simulink model "speed_modelo_motor_frenado_con_codigoC"  (R2022b)
settings: Solver=VariableStepAuto  StartTime=0.0  StopTime=5  FixedStep=0.01  MaxStep=0.00005  RelTol=1e-3
undefined symbols (not defined in the file): frec_max_f_freno, frec_motor_max_f, frecuencia, frecuencia_freno, FuerzaX_acel, FuerzaX_freno, FuerzaY_acel, Ipeak, L, mass, pole_length, r, slip, slip_freno, vel_motor_max_f, vel_motor_max_f_freno
libraries: slpidlib x2, pi_con_C x1, eePowerMeasurement x1
settings Model: Creator=mique  LastModifiedBy=mique
settings SolverCC: ZeroCrossAlgorithm=Adaptive
settings DebuggingCC: IgnoredZcDiagnostic=none

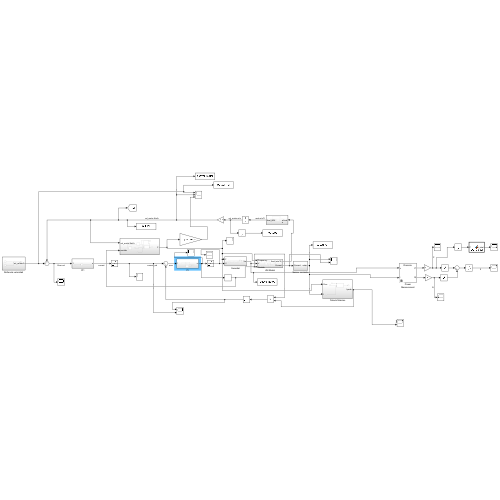
[thumbnail: Simulink's stored preview of the top-level diagram]
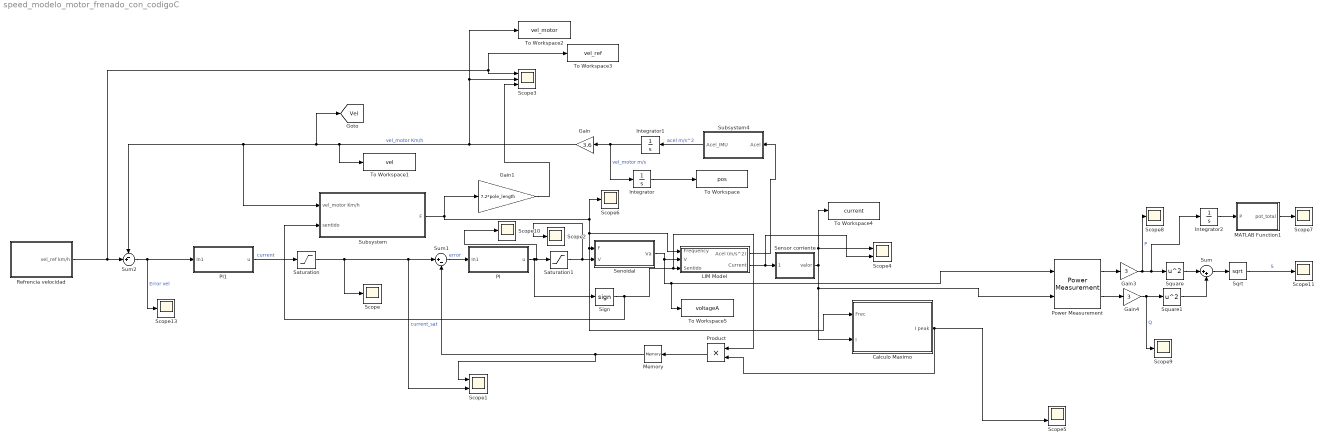
== system speed_modelo_motor_frenado_con_codigoC ==
  Calculo Maximo : Subsystem
  Gain : Gain  Gain=3.6
  Gain1 : Gain  Gain=7.2*pole_length
  Gain3 : Gain  Gain=3
  Gain4 : Gain  Gain=3
  Integrator : Integrator
  Integrator1 : Integrator
  Integrator2 : Integrator
  LIM Model : Subsystem
  MATLAB Function1 : MATLAB Function  TreatAsAtomicUnit=on
  Memory : Memory
  PI : Subsystem
  PI1 : Subsystem
  Power Measurement : eePowerMeasurement/Power Measurement  LabelModeActiveChoice=Discrete  F=8  K=[0 1 2 3 4 5 6 7 8 9 10 11]  Ts=0.0002
  Product : Product
  Refrencia velocidad : Subsystem
  Saturation : Saturate  UpperLimit=100  LowerLimit=-100
  Saturation1 : Saturate  UpperLimit=200  LowerLimit=-200
  Scope{,2,6..11,13} (9 alike) : Scope
  Scope1 : Scope  NumInputPorts=2
  Scope3 : Scope  NumInputPorts=3
  Scope4 : Scope  NumInputPorts=2
  Scope5 : Scope  NumInputPorts=2
  Senoidal : Subsystem
  Sensor corriente : Subsystem
  Sign : Signum
  Sqrt : Sqrt
  Square : Math  Operator=square
  Square1 : Math  Operator=square
  Subsystem : Subsystem
  Subsystem4 : Subsystem
  Sum : Sum  Inputs=|++
  Sum1 : Sum  Inputs=|+-
  Sum2 : Sum  Inputs=-+|
  To Workspace : ToWorkspace  VariableName=pos  SampleTime=-1
  To Workspace1 : ToWorkspace  VariableName=vel  SampleTime=-1
  To Workspace2 : ToWorkspace  VariableName=vel_motor  SampleTime=-1
  To Workspace3 : ToWorkspace  VariableName=vel_ref  SampleTime=-1
  To Workspace4 : ToWorkspace  VariableName=current  SampleTime=-1
  To Workspace5 : ToWorkspace  VariableName=voltageA  SaveFormat=Timeseries  SampleTime=-1
  tag scope: Vel=global
  wires:
  Integrator1/1 -> Integrator/1, Gain/1  "vel_motor m/s"
  Gain/1 -> To Workspace2/1, Scope3/2, To Workspace1/1, [Vel], Subsystem/1(vel_motor Km/h), Sum2/1  "vel_motor Km/h"
  LIM Model/1(Acel (m/s^2)) -> Subsystem4/1(Acel)
  Integrator/1 -> To Workspace/1
  Sum1/1 -> PI/1(In1)  "error"
  Sum2/1 -> PI1/1(In1), Scope13/1  "Error vel"
  Refrencia velocidad/1(vel_ref km/h) -> To Workspace3/1, Scope3/1, Sum2/2
  PI1/1(u) -> Saturation/1  "current"
  Gain1/1 -> Scope3/3
  Saturation/1 -> Scope/1, Scope1/2, Sum1/1  "current_sat"
  Subsystem4/1(Acel_IMU) -> Integrator1/1  "acel m/s^2"
  LIM Model/2(Current) -> Scope4/2, Sensor corriente/1(Current)
  Senoidal/1(Va) -> To Workspace5/1, Power Measurement/1, LIM Model/2("V ")
  Power Measurement/1 -> Gain3/1
  Gain3/1 -> Integrator2/1, Square/1, Scope8/1  "P"
  Power Measurement/2 -> Gain4/1
  Gain4/1 -> Scope9/1, Square1/1  "Q"
  Square/1 -> Sum/1
  Square1/1 -> Sum/2
  Sum/1 -> Sqrt/1
  Sqrt/1 -> Scope11/1  "S"
  Sign/1 -> Subsystem/2(sentido), Product/1, LIM Model/3(Sentido)
  Product/1 -> Memory/1
  Memory/1 -> Scope1/1, Sum1/2
  Sensor corriente/1(valor) -> To Workspace4/1, Scope4/1, Calculo Maximo/2(I), Power Measurement/2
  PI/1(u) -> Sign/1, Scope10/1, Saturation1/1
  Saturation1/1 -> Scope2/1, Senoidal/2(V)
  Integrator2/1 -> MATLAB Function1/1(P)
  MATLAB Function1/1(pot_total) -> Scope7/1
  Subsystem/1(F) -> Gain1/1, Scope6/1, Calculo Maximo/1(Frec), Senoidal/1(F), LIM Model/1(Frequency)
  Calculo Maximo/1(I peak) -> Product/2, Scope5/2

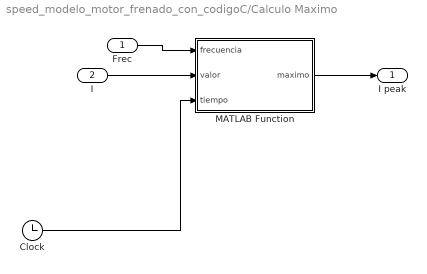
== system speed_modelo_motor_frenado_con_codigoC/Calculo Maximo ==
  Frec : Inport
  I : Inport  Port=2
  Clock : Clock
  MATLAB Function : MATLAB Function  TreatAsAtomicUnit=on
  I peak : Outport
  wires:
  Frec/1 -> MATLAB Function/1(frecuencia)
  I/1 -> MATLAB Function/2(valor)
  MATLAB Function/1(maximo) -> I peak/1
  Clock/1 -> MATLAB Function/3(tiempo)

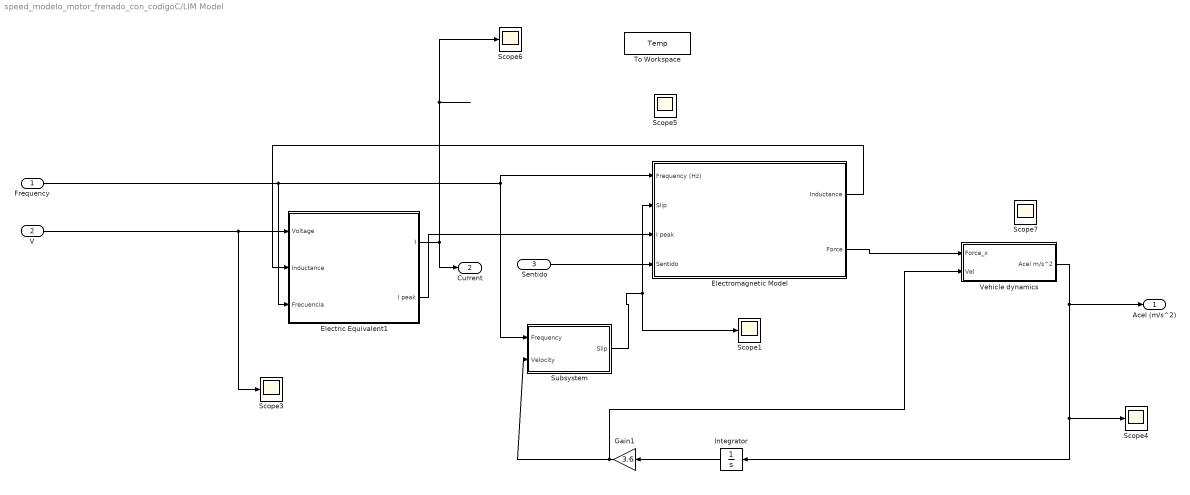
== system speed_modelo_motor_frenado_con_codigoC/LIM Model ==
  Frequency : Inport
  "V " : Inport  Port=2
  Sentido : Inport  Port=3
  Electric Equivalent1 : Subsystem
  Electromagnetic Model : Subsystem
  Gain1 : Gain  Gain=3.6
  Integrator : Integrator
  Scope{1,3..7} (6 alike) : Scope
  Subsystem : Subsystem
  To Workspace : ToWorkspace  VariableName=Temp  SampleTime=-1
  Vehicle dynamics : Subsystem
  Acel (m/s^2) : Outport
  Current : Outport  Port=2
  wires:
  Vehicle dynamics/1(Acel m/s^2) -> Integrator/1, Scope4/1, Acel (m/s^2)/1
  Electric Equivalent1/2(I peak) -> Electromagnetic Model/3(I peak)
  Electromagnetic Model/1(Inductance) -> Electric Equivalent1/2(Inductance)
  Frequency/1 -> Electric Equivalent1/3(Frecuencia), Subsystem/1(Frequency), Electromagnetic Model/1(Frequency (Hz))
  Integrator/1 -> Gain1/1
  "V "/1 -> Scope3/1, Electric Equivalent1/1(Voltage)
  ? -> Scope5/1, To Workspace/1
  Electric Equivalent1/1("I ") -> Current/1, Scope6/1
  Sentido/1 -> Electromagnetic Model/4(Sentido)
  Subsystem/1(Slip) -> Scope1/1, Electromagnetic Model/2(Slip)
  Gain1/1 -> Vehicle dynamics/2(Vel), Subsystem/2(Velocity)
  Electromagnetic Model/2(Force) -> Vehicle dynamics/1(Force_x)

== system speed_modelo_motor_frenado_con_codigoC/PI ==
  note: Parametros obtenidos con el PID tuner
  In1 : Inport
  Discrete PID Controller1 : slpidlib/PID Controller  Controller=PI  Form=Parallel  TimeDomain=Discrete-time  UseExternalTs=off  SampleTime=0.0002  IntegratorMethod=Forward Euler  FilterMethod=Forward Euler  ControllerParametersSource=internal  P=0.3  I=5  UseKiTs=off  D=0.5  N=10  UseFilter=on  TunerSelectOption=Transfer Function Based (PID Tuner App)  InitialConditionSource=internal  InitialConditionForIntegrator=0  InitialConditionForFilter=0  DifferentiatorICPrevScaledInput=0  ExternalReset=none  TrackingMode=off  Kt=1  LimitOutput=off  SatLimitsSource=internal  UpperSaturationLimit=100  LowerSaturationLimit=-inf  LinearizeAsGain=off  AntiWindupMode=back-calculation  Kb=1  LimitIntegrator=off  UpperIntegratorSaturationLimit=15  LowerIntegratorSaturationLimit=-15  POutMin=[]  POutMax=[]  IOutMin=[]  IOutMax=[]  DOutMin=[]  DOutMax=[]  NOutMin=[]  NOutMax=[]  SumOutMin=[]  SumOutMax=[]  SaturationOutMin=[]  SaturationOutMax=[]  PParamMin=[]  PParamMax=[]  IParamMin=[]  IParamMax=[]  DParamMin=[]  DParamMax=[]  NParamMin=[]  NParamMax=[]  KbParamMin=[]  KbParamMax=[]  KtParamMin=[]  KtParamMax=[]  KbOutMin=[]  KbOutMax=[]  KtOutMin=[]  KtOutMax=[]  IntegratorOutMin=[]  IntegratorOutMax=[]  FilterOutMin=[]  FilterOutMax=[]  SumI1OutMin=[]  SumI1OutMax=[]  SumI2OutMin=[]  SumI2OutMax=[]  SumI3OutMin=[]  SumI3OutMax=[]  SumI4OutMin=[]  SumI4OutMax=[]  SumDOutMin=[]  SumDOutMax=[]  DifferentiatorOutMin=[]  DifferentiatorOutMax=[]  FilterDiffOutCoefMin=[]  FilterDiffOutCoefMax=[]  ReciprocalOutMin=[]  ReciprocalOutMax=[]  SumDenOutMin=[]  SumDenOutMax=[]  SumNumOutMin=[]  SumNumOutMax=[]  DivideOutMin=[]  DivideOutMax=[]  UdiffTsProdOutMin=[]  UdiffTsProdOutMax=[]  NTsProdOutMin=[]  NTsProdOutMax=[]  UintegralTsProdOutMin=[]  UintegralTsProdOutMax=[]  UngainTsProdOutMin=[]  UngainTsProdOutMax=[]  ClampingZeroOutDataTypeStr=Inherit: Inherit via back propagation  ClampingZeroOutMin=[]  ClampingZeroOutMax=[]  FilterDenConstantOutDataTypeStr=Inherit: Inherit via back propagation  FilterDenConstantOutMin=[]  FilterDenConstantOutMax=[]  PCopyOutDataTypeStr=Inherit: Inherit via back propagation  PCopyOutMin=[]  PCopyOutMax=[]  NCopyOutDataTypeStr=Inherit: Inherit via back propagation  NCopyOutMin=[]  NCopyOutMax=[]  IntegratorContinuousStateAttributes=''  IntegratorStateMustResolveToSignalObject=off  IntegratorRTWStateStorageClass=Auto  FilterContinuousStateAttributes=''  FilterStateMustResolveToSignalObject=off  FilterRTWStateStorageClass=Auto  ParallelPVariant=InternalParameters  IdealPVariant=Disabled  IVariant=InternalParameters  DVariant=Disabled  IntegratorVariant=Discrete  SatVariant=Disabled  AWVariant=Passthrough  PCopyVariant=Disabled  TRVariant=Disabled  FdbkBlocksVariant=Forward  IdealPFdbkVariant=Disabled  SatFdbkVariant=Disabled  DerivativeFilterVariant=Disabled  NVariant=Disabled  NCopyVariant=Disabled_SignalSpec  FilterICVariant=Disabled  IntegratorICVariant=InternalICs  ExternalResetVariant=Disabled  TRSumVariant=Passthrough  SumFdbkVariant=Disabled  SumVariant=Sum_PI  TsampFilterVariant=InternalTs  TsampNgainVariant=Passthrough  TsampIntegralVariant=Passthrough  ExternalSaturationOutDataTypeStr=Inherit: Same as second input
      settings: LibrarySourceBlock=simulink/Discrete/Discrete PID Controller
  PI_controller : pi_con_C/PI_controller  SampleTime=0.0002
  Scope : Scope  NumInputPorts=2
  u : Outport
  wires:
  In1/1 -> PI_controller/1, Discrete PID Controller1/1
  Discrete PID Controller1/1 -> Scope/1, u/1
  PI_controller/1 -> Scope/2

== system speed_modelo_motor_frenado_con_codigoC/PI1 ==
  note: Parametros obtenidos con el PID tuner
  In1 : Inport
  Discrete PID Controller1 : slpidlib/PID Controller  Controller=PI  Form=Parallel  TimeDomain=Discrete-time  UseExternalTs=off  SampleTime=0.001  IntegratorMethod=Forward Euler  FilterMethod=Forward Euler  ControllerParametersSource=internal  P=40  I=15  UseKiTs=off  D=0.2  N=10  UseFilter=on  TunerSelectOption=Transfer Function Based (PID Tuner App)  InitialConditionSource=internal  InitialConditionForIntegrator=0  InitialConditionForFilter=0  DifferentiatorICPrevScaledInput=0  ExternalReset=none  TrackingMode=off  Kt=1  LimitOutput=off  SatLimitsSource=internal  UpperSaturationLimit=100  LowerSaturationLimit=-100  LinearizeAsGain=off  AntiWindupMode=clamping  Kb=0.1  LimitIntegrator=on  UpperIntegratorSaturationLimit=15  LowerIntegratorSaturationLimit=-15  POutMin=[]  POutMax=[]  IOutMin=[]  IOutMax=[]  DOutMin=[]  DOutMax=[]  NOutMin=[]  NOutMax=[]  SumOutMin=[]  SumOutMax=[]  SaturationOutMin=[]  SaturationOutMax=[]  PParamMin=[]  PParamMax=[]  IParamMin=[]  IParamMax=[]  DParamMin=[]  DParamMax=[]  NParamMin=[]  NParamMax=[]  KbParamMin=[]  KbParamMax=[]  KtParamMin=[]  KtParamMax=[]  KbOutMin=[]  KbOutMax=[]  KtOutMin=[]  KtOutMax=[]  IntegratorOutMin=[]  IntegratorOutMax=[]  FilterOutMin=[]  FilterOutMax=[]  SumI1OutMin=[]  SumI1OutMax=[]  SumI2OutMin=[]  SumI2OutMax=[]  SumI3OutMin=[]  SumI3OutMax=[]  SumI4OutMin=[]  SumI4OutMax=[]  SumDOutMin=[]  SumDOutMax=[]  DifferentiatorOutMin=[]  DifferentiatorOutMax=[]  FilterDiffOutCoefMin=[]  FilterDiffOutCoefMax=[]  ReciprocalOutMin=[]  ReciprocalOutMax=[]  SumDenOutMin=[]  SumDenOutMax=[]  SumNumOutMin=[]  SumNumOutMax=[]  DivideOutMin=[]  DivideOutMax=[]  UdiffTsProdOutMin=[]  UdiffTsProdOutMax=[]  NTsProdOutMin=[]  NTsProdOutMax=[]  UintegralTsProdOutMin=[]  UintegralTsProdOutMax=[]  UngainTsProdOutMin=[]  UngainTsProdOutMax=[]  ClampingZeroOutDataTypeStr=Inherit: Inherit via back propagation  ClampingZeroOutMin=[]  ClampingZeroOutMax=[]  FilterDenConstantOutDataTypeStr=Inherit: Inherit via back propagation  FilterDenConstantOutMin=[]  FilterDenConstantOutMax=[]  PCopyOutDataTypeStr=Inherit: Inherit via back propagation  PCopyOutMin=[]  PCopyOutMax=[]  NCopyOutDataTypeStr=Inherit: Inherit via back propagation  NCopyOutMin=[]  NCopyOutMax=[]  IntegratorContinuousStateAttributes=''  IntegratorStateMustResolveToSignalObject=off  IntegratorRTWStateStorageClass=Auto  FilterContinuousStateAttributes=''  FilterStateMustResolveToSignalObject=off  FilterRTWStateStorageClass=Auto  ParallelPVariant=InternalParameters  IdealPVariant=Disabled  IVariant=InternalParameters  DVariant=Disabled  IntegratorVariant=Discrete  SatVariant=Disabled  AWVariant=Passthrough  PCopyVariant=Disabled  TRVariant=Disabled  FdbkBlocksVariant=Forward  IdealPFdbkVariant=Disabled  SatFdbkVariant=Disabled  DerivativeFilterVariant=Disabled  NVariant=Disabled  NCopyVariant=Disabled_SignalSpec  FilterICVariant=Disabled  IntegratorICVariant=InternalICs  ExternalResetVariant=Disabled  TRSumVariant=Passthrough  SumFdbkVariant=Disabled  SumVariant=Sum_PI  TsampFilterVariant=InternalTs  TsampNgainVariant=Passthrough  TsampIntegralVariant=Passthrough  ExternalSaturationOutDataTypeStr=Inherit: Same as second input
      settings: LibrarySourceBlock=simulink/Discrete/Discrete PID Controller
  u : Outport
  wires:
  Discrete PID Controller1/1 -> u/1
  In1/1 -> Discrete PID Controller1/1

== system speed_modelo_motor_frenado_con_codigoC/Refrencia velocidad ==
  Step : Step  Time=0.5  After=35  SampleTime=0
  Step1 : Step  Time=2.5  After=-35  SampleTime=0
  Sum : Sum  Inputs=|++
  vel_ref km/h : Outport
  wires:
  Step/1 -> Sum/1
  Step1/1 -> Sum/2
  Sum/1 -> vel_ref km/h/1

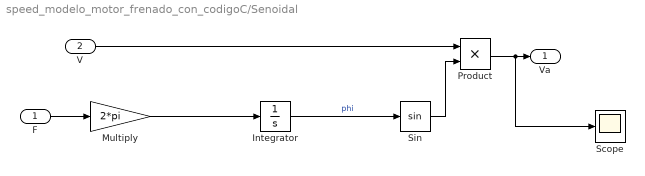
== system speed_modelo_motor_frenado_con_codigoC/Senoidal ==
  F : Inport
  V : Inport  Port=2
  Integrator : Integrator  WrapState=on  WrappedStateUpperValue=2*pi  WrappedStateLowerValue=0
  Multiply : Gain  Gain=2*pi
  Product : Product
  Scope : Scope
  Sin : Trigonometry
  Va : Outport
  wires:
  Integrator/1 -> Sin/1  "phi"
  V/1 -> Product/1
  Sin/1 -> Product/2
  Product/1 -> Scope/1, Va/1
  F/1 -> Multiply/1
  Multiply/1 -> Integrator/1

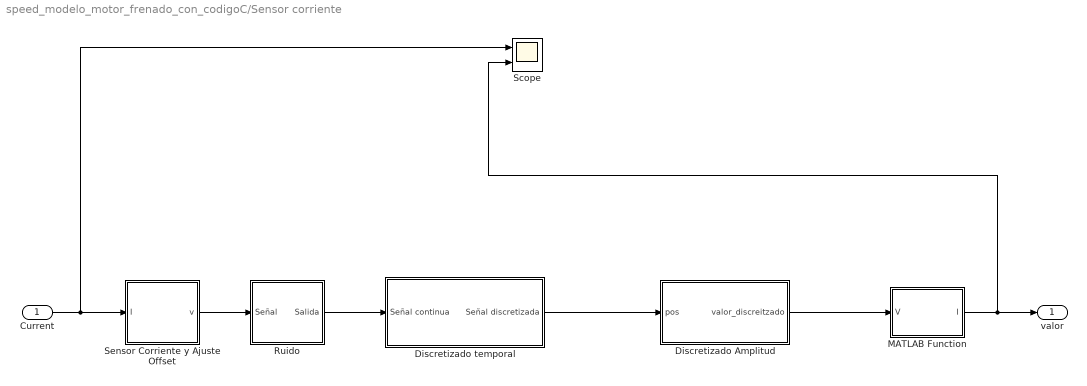
== system speed_modelo_motor_frenado_con_codigoC/Sensor corriente ==
  Current : Inport
  Discretizado Amplitud : Subsystem  mask{Num_Val=1000, Max=4, Min=1}
      mask prompts: Num_Val "Numero de valores distintos"; Max "Maximo valor"; Min "Minimo valor"
  Discretizado temporal : Subsystem  mask{Tiempo_Discretizado=0.0002}
      mask prompts: Tiempo_Discretizado "Tiempo de discretizacion (s)"
      mask DialogControl DescGroupVar Prompt: Discretiza una señal mediante un ZOH con un tiempo definido
  MATLAB Function : MATLAB Function  TreatAsAtomicUnit=on
  Ruido : Subsystem  mask{M=0, V=0.0001, f=50}
      mask prompts: M "Media"; V "Varianza"; f "Frecuencia (Hz)"
      mask init:
      | T=1/f;
      mask DialogControl DescGroupVar Prompt: Añadidor de Ruido
      mask DialogControl DescTextVar Prompt: Añade un ruido blanco Gausiano con los siguientes valores:
  Scope : Scope  NumInputPorts=2
  Sensor Corriente y Ajuste Offset : Subsystem  mask{offset=0.001, max=off}
      mask prompts: max "Offset positivo"
      mask init:
      | if(max==true)
      |         offset=abs(offset);
      | 
      |     else
      |         offset=-offset;
      |     end
  valor : Outport
  wires:
  Discretizado Amplitud/1(valor_discreitzado) -> MATLAB Function/1(V)
  Discretizado temporal/1(Señal discretizada) -> Discretizado Amplitud/1(pos)
  Sensor Corriente y Ajuste Offset/1(v) -> Ruido/1(Señal)
  Ruido/1(Salida) -> Discretizado temporal/1(Señal continua)
  Current/1 -> Scope/1, Sensor Corriente y Ajuste Offset/1(I)
  MATLAB Function/1(I) -> Scope/2, valor/1

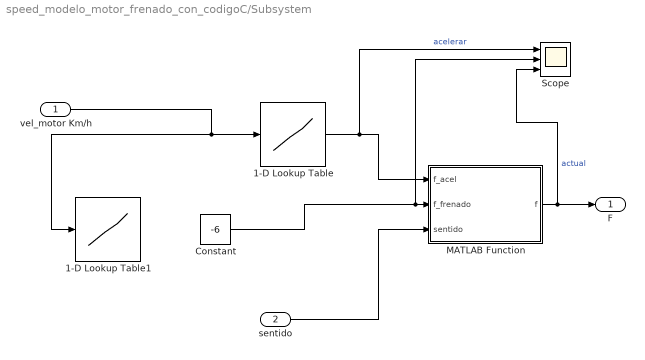
== system speed_modelo_motor_frenado_con_codigoC/Subsystem ==
  vel_motor Km/h : Inport
  sentido : Inport  Port=2
  1-D Lookup Table : Lookup_n-D  NumberOfTableDimensions=1  BreakpointsForDimension1=vel_motor_max_f  Table=frec_motor_max_f  InternalRulePriority=Speed  RndMeth=Simplest
  1-D Lookup Table1 : Lookup_n-D  NumberOfTableDimensions=1  BreakpointsForDimension1=vel_motor_max_f_freno  Table=frec_max_f_freno  InternalRulePriority=Speed  RndMeth=Simplest
  Constant : Constant  Value=-6
  MATLAB Function : MATLAB Function  TreatAsAtomicUnit=on
  Scope : Scope  NumInputPorts=3
  F : Outport
  wires:
  vel_motor Km/h/1 -> 1-D Lookup Table/1, 1-D Lookup Table1/1
  sentido/1 -> MATLAB Function/3(sentido)
  1-D Lookup Table/1 -> Scope/1, MATLAB Function/1(f_acel)  "acelerar"
  MATLAB Function/1(f) -> Scope/3, F/1  "actual"
  Constant/1 -> Scope/2, MATLAB Function/2(f_frenado)

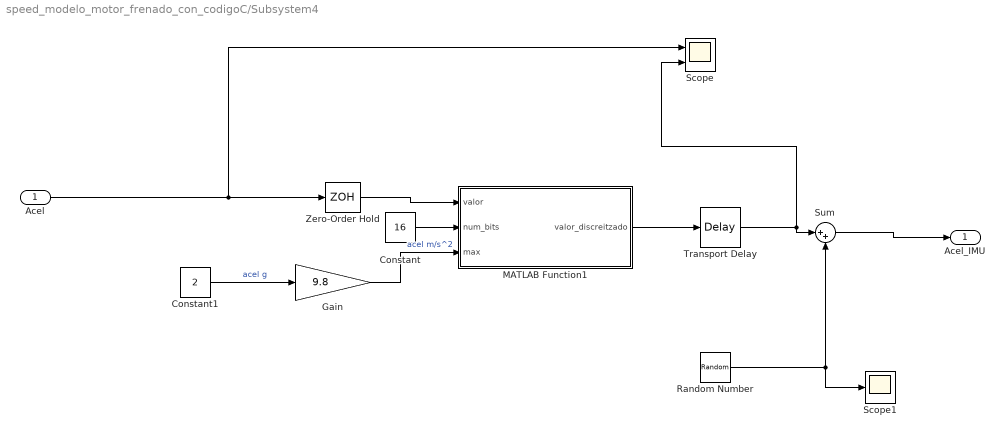
== system speed_modelo_motor_frenado_con_codigoC/Subsystem4 ==
  Acel : Inport
  Constant : Constant  Value=16
  Constant1 : Constant  Value=2
  Gain : Gain  Gain=9.8
  MATLAB Function1 : MATLAB Function  TreatAsAtomicUnit=on
  Random Number : RandomNumber  Variance=0.1  SampleTime=0.001
  Scope : Scope  NumInputPorts=2
  Scope1 : Scope
  Sum : Sum  Inputs=|++
  Transport Delay : TransportDelay  DelayTime=0.001
  Zero-Order Hold : ZeroOrderHold  SampleTime=0.001
  Acel_IMU : Outport
  wires:
  MATLAB Function1/1(valor_discreitzado) -> Transport Delay/1
  Zero-Order Hold/1 -> MATLAB Function1/1(valor)
  Constant1/1 -> Gain/1  "acel g"
  Constant/1 -> MATLAB Function1/2(num_bits)
  Gain/1 -> MATLAB Function1/3(max)  "acel m/s^2"
  Transport Delay/1 -> Sum/1, Scope/2
  Acel/1 -> Scope/1, Zero-Order Hold/1
  Sum/1 -> Acel_IMU/1
  Random Number/1 -> Scope1/1, Sum/2

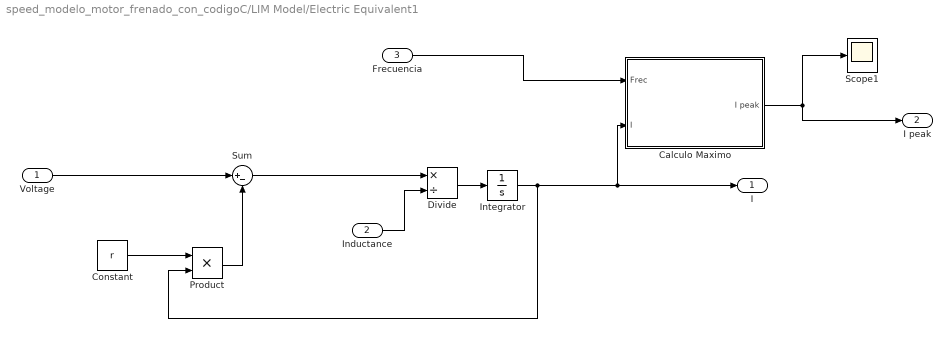
== system speed_modelo_motor_frenado_con_codigoC/LIM Model/Electric Equivalent1 ==
  Voltage : Inport
  Inductance : Inport  Port=2
  Frecuencia : Inport  Port=3
  Calculo Maximo : Subsystem
  Constant : Constant  Value=r
  Divide : Product  Inputs=*/
  Integrator : Integrator
  Product : Product
  Scope1 : Scope
  Sum : Sum  Inputs=|+-
  "I " : Outport
  I peak : Outport  Port=2
  wires:
  Voltage/1 -> Sum/1
  Integrator/1 -> Calculo Maximo/2(I), "I "/1, Product/2
  Constant/1 -> Product/1
  Product/1 -> Sum/2
  Divide/1 -> Integrator/1
  Sum/1 -> Divide/1
  Inductance/1 -> Divide/2
  Calculo Maximo/1(I peak) -> I peak/1, Scope1/1
  Frecuencia/1 -> Calculo Maximo/1(Frec)

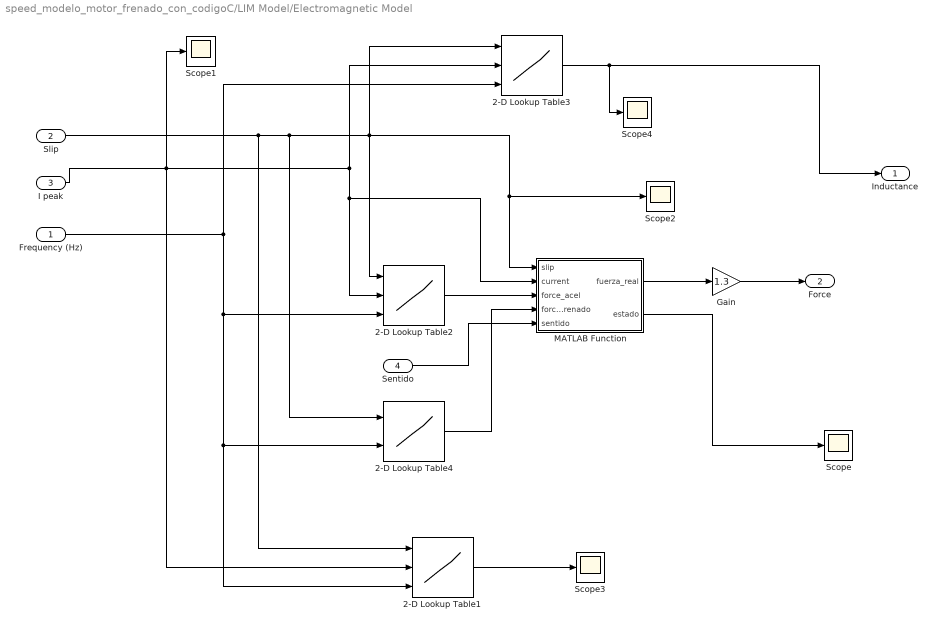
== system speed_modelo_motor_frenado_con_codigoC/LIM Model/Electromagnetic Model ==
  Frequency (Hz) : Inport
  Slip : Inport  Port=2
  I peak : Inport  Port=3
  Sentido : Inport  Port=4
  2-D Lookup Table1 : Lookup_n-D  NumberOfTableDimensions=3  BreakpointsForDimension1=slip  BreakpointsForDimension2=Ipeak  BreakpointsForDimension3=frecuencia  Table=FuerzaY_acel  InterpMethod=Nearest  InternalRulePriority=Speed  RndMeth=Simplest
      settings: InputPortMap=u0,u1,u2
  2-D Lookup Table2 : Lookup_n-D  NumberOfTableDimensions=3  BreakpointsForDimension1=slip  BreakpointsForDimension2=Ipeak  BreakpointsForDimension3=frecuencia  Table=FuerzaX_acel  InterpMethod=Nearest  InternalRulePriority=Speed  RndMeth=Simplest
      settings: InputPortMap=u0,u1,u2
  2-D Lookup Table3 : Lookup_n-D  NumberOfTableDimensions=3  BreakpointsForDimension1=Ipeak(2:(end-1))  BreakpointsForDimension2=slip  BreakpointsForDimension3=frecuencia  Table=L  InterpMethod=Nearest  InternalRulePriority=Speed  RndMeth=Simplest
      settings: InputPortMap=u0,u1,u2
  2-D Lookup Table4 : Lookup_n-D  BreakpointsForDimension1=slip_freno  BreakpointsForDimension2=frecuencia_freno  BreakpointsForDimension3=frecuencia  Table=FuerzaX_freno  InterpMethod=Nearest  InternalRulePriority=Speed  RndMeth=Simplest
      settings: InputPortMap=u0,u1
  Gain : Gain  Gain=1.3
  MATLAB Function : MATLAB Function  TreatAsAtomicUnit=on
  Scope{,1..4} (5 alike) : Scope
  Inductance : Outport
  Force : Outport  Port=2
  wires:
  2-D Lookup Table3/1 -> Scope4/1, Inductance/1
  Frequency (Hz)/1 -> 2-D Lookup Table4/2, 2-D Lookup Table1/3, 2-D Lookup Table2/3, 2-D Lookup Table3/3
  I peak/1 -> 2-D Lookup Table1/2, MATLAB Function/2(current), 2-D Lookup Table2/2, 2-D Lookup Table3/2, Scope1/1
  Slip/1 -> 2-D Lookup Table1/1, 2-D Lookup Table4/1, Scope2/1, MATLAB Function/1(slip), 2-D Lookup Table2/1, 2-D Lookup Table3/1
  2-D Lookup Table2/1 -> MATLAB Function/3(force_acel)
  2-D Lookup Table1/1 -> Scope3/1
  2-D Lookup Table4/1 -> MATLAB Function/4(force_frenado)
  Sentido/1 -> MATLAB Function/5(sentido)
  MATLAB Function/2(estado) -> Scope/1
  MATLAB Function/1(fuerza_real) -> Gain/1
  Gain/1 -> Force/1

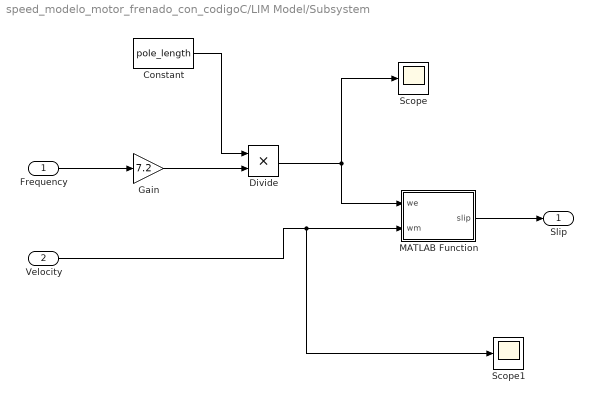
== system speed_modelo_motor_frenado_con_codigoC/LIM Model/Subsystem ==
  Frequency : Inport
  Velocity : Inport  Port=2
  Constant : Constant  Value=pole_length
  Divide : Product  Inputs=**
  Gain : Gain  Gain=7.2
  MATLAB Function : MATLAB Function  TreatAsAtomicUnit=on
  Scope : Scope
  Scope1 : Scope
  Slip : Outport
  wires:
  Frequency/1 -> Gain/1
  MATLAB Function/1(slip) -> Slip/1
  Gain/1 -> Divide/2
  Constant/1 -> Divide/1
  Divide/1 -> Scope/1, MATLAB Function/1(we)
  Velocity/1 -> Scope1/1, MATLAB Function/2(wm)

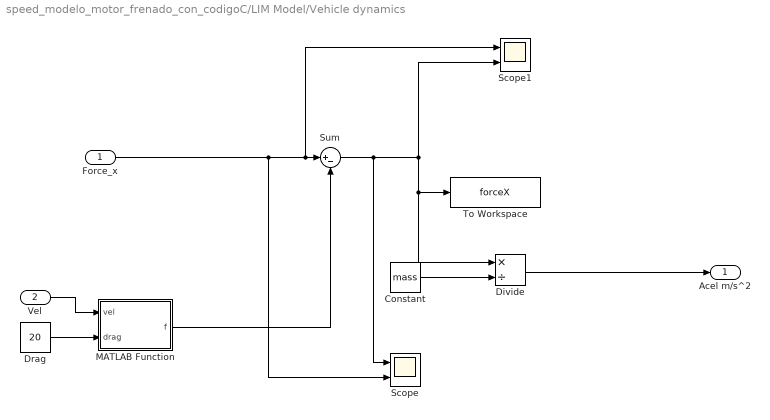
== system speed_modelo_motor_frenado_con_codigoC/LIM Model/Vehicle dynamics ==
  Force_x : Inport
  Vel : Inport  Port=2
  Constant : Constant  Value=mass
  Divide : Product  Inputs=*/
  Drag : Constant  Value=20
  MATLAB Function : MATLAB Function  TreatAsAtomicUnit=on
  Scope : Scope  NumInputPorts=2
  Scope1 : Scope  NumInputPorts=2
  Sum : Sum  Inputs=|+-
  To Workspace : ToWorkspace  VariableName=forceX  SampleTime=-1
  Acel m/s^2 : Outport
  wires:
  Divide/1 -> Acel m/s^2/1
  Constant/1 -> Divide/2
  Force_x/1 -> Scope/2, Scope1/1, Sum/1
  Sum/1 -> Scope/1, Scope1/2, Divide/1, To Workspace/1
  Drag/1 -> MATLAB Function/2(drag)
  Vel/1 -> MATLAB Function/1(vel)
  MATLAB Function/1(f) -> Sum/2

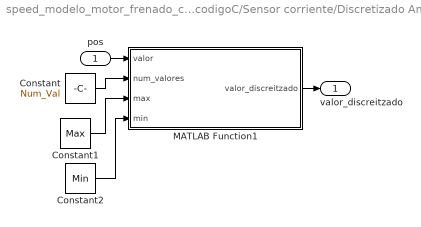
== system speed_modelo_motor_frenado_con_codigoC/Sensor corriente/Discretizado Amplitud ==
  pos : Inport
  Constant : Constant  Value=Num_Val
  Constant1 : Constant  Value=Max
  Constant2 : Constant  Value=Min
  MATLAB Function1 : MATLAB Function  TreatAsAtomicUnit=on
  valor_discreitzado : Outport
  wires:
  pos/1 -> MATLAB Function1/1(valor)
  Constant2/1 -> MATLAB Function1/4(min)
  Constant/1 -> MATLAB Function1/2(num_valores)
  Constant1/1 -> MATLAB Function1/3(max)
  MATLAB Function1/1(valor_discreitzado) -> valor_discreitzado/1

== system speed_modelo_motor_frenado_con_codigoC/Sensor corriente/Discretizado temporal ==
  Señal continua : Inport
  Zero-Order Hold : ZeroOrderHold  SampleTime=Tiempo_Discretizado
  Señal discretizada : Outport
  wires:
  Zero-Order Hold/1 -> Señal discretizada/1
  Señal continua/1 -> Zero-Order Hold/1

== system speed_modelo_motor_frenado_con_codigoC/Sensor corriente/Ruido ==
  Señal : Inport
  Ruido : RandomNumber  Mean=M  Variance=V  Seed=10  SampleTime=T
  Sum : Sum  Inputs=|++
  Salida : Outport
  wires:
  Sum/1 -> Salida/1
  Ruido/1 -> Sum/1
  Señal/1 -> Sum/2

== system speed_modelo_motor_frenado_con_codigoC/Sensor corriente/Sensor Corriente y Ajuste Offset ==
  I : Inport
  Constant : Constant  Value=offset
  Sensor : MATLAB Function  TreatAsAtomicUnit=on
  v : Outport
  wires:
  I/1 -> Sensor/1(I)
  Constant/1 -> Sensor/2(offset)
  Sensor/1(V_o) -> v/1

== system speed_modelo_motor_frenado_con_codigoC/LIM Model/Electric Equivalent1/Calculo Maximo ==
  Frec : Inport
  I : Inport  Port=2
  Clock : Clock
  MATLAB Function : MATLAB Function  TreatAsAtomicUnit=on
  I peak : Outport
  wires:
  Frec/1 -> MATLAB Function/1(frecuencia)
  I/1 -> MATLAB Function/2(valor)
  MATLAB Function/1(maximo) -> I peak/1
  Clock/1 -> MATLAB Function/3(tiempo)

== matlab function speed_modelo_motor_frenado_con_codigoC/LIM Model/Electromagnetic Model/MATLAB Function ==
  data: slip input; fuerza_real output; current input; force_acel input; force_frenado input; sentido input; estado output
function [fuerza_real,estado]= fcn(slip,current,force_acel,force_frenado,sentido)

if sentido>=0
    force=force_acel;
    estado=1;
else
    force=force_frenado;
    estado=2;
end

if slip == 0 || current<2 && current>-2

    fuerza_real=0;
    estado=3;

else
    fuerza_real=force;
    estado=4;
end

== matlab function speed_modelo_motor_frenado_con_codigoC/Sensor corriente/Discretizado Amplitud/MATLAB Function1 ==
  data: valor input; valor_discreitzado output; num_valores input; max input; min input
function valor_discreitzado  = fcn(valor,num_valores,max,min)

if(valor>max)
    valor_discreitzado=max;
    return
end
if(valor<min)
    valor_discreitzado=min;
    return
end


valor_escalon=(max-min)/(num_valores-1);


i=min;
 while(i<max)
    if(i+valor_escalon/2>valor)
        valor_discreitzado=i;
        return
    end
    i=i+valor_escalon;
end



      valor_discreitzado=max;
end

== matlab function speed_modelo_motor_frenado_con_codigoC/LIM Model/Electric Equivalent1/Calculo Maximo/MATLAB Function ==
  settings: updateMethod=DISCRETE
  data: frecuencia input; maximo output; valor input; tiempo input
function maximo = fcn(frecuencia,valor,tiempo)

   persistent antiguo_maximo
    if isempty(antiguo_maximo)
       antiguo_maximo=0;
    end
    persistent t_maximo
    if isempty(t_maximo)
       t_maximo=0;
    end

periodo=1/abs(frecuencia);


if abs(valor)>=antiguo_maximo
    maximo=abs(valor);
    antiguo_maximo=abs(valor);
    t_maximo=tiempo;
else
    maximo=antiguo_maximo;
    if tiempo>t_maximo+periodo
        maximo=abs(valor);
        antiguo_maximo=abs(valor);
        t_maximo=tiempo;
    end
end

== matlab function speed_modelo_motor_frenado_con_codigoC/LIM Model/Subsystem/MATLAB Function ==
  data: we input; slip output; wm input
function slip = fcn(we,wm)

slip = (we-wm)/we;

== matlab function speed_modelo_motor_frenado_con_codigoC/Subsystem/MATLAB Function ==
  data: f_acel input; f output; f_frenado input; sentido input
function f= fcn(f_acel,f_frenado,sentido)

if sentido>=0
    f=f_acel;

else
    f=f_frenado;

end

== matlab function speed_modelo_motor_frenado_con_codigoC/MATLAB Function1 ==
  data: P input; pot_total output
function pot_total = efecto_total(P)

pot_total=0;
for k=1:max(size(P))
    pot_total=pot_total+P(k);
end

== matlab function speed_modelo_motor_frenado_con_codigoC/Sensor corriente/MATLAB Function ==
  data: V input; I output
function I = fcn(V)

I=(V-2.5)/0.005;

== matlab function speed_modelo_motor_frenado_con_codigoC/Subsystem4/MATLAB Function1 ==
  data: valor input; valor_discreitzado output; num_bits input; max input
function valor_discreitzado  = fcn(valor,num_bits,max)

min=-max;
num_valores=2^num_bits;
if(valor>max)
    valor_discreitzado=max;
    return
end
if(valor<min)
    valor_discreitzado=min;
    return
end


valor_escalon=(max-min)/(num_valores-1);


i=min;
 while(i<max)
    if(i+valor_escalon/2>valor)
        valor_discreitzado=i;
        return
    end
    i=i+valor_escalon;
end



      valor_discreitzado=max;
end

== matlab function speed_modelo_motor_frenado_con_codigoC/Sensor corriente/Sensor Corriente y Ajuste Offset/Sensor ==
  data: I input; V_o output; offset input
function V_o = Sensor_L01Z300S05(I,offset)
Vcc=5;
if(I>300)
    I=300;
end
if(I<-300)
    I=-300;
end
V_ref=Vcc/2;
V_o=V_ref+0.005*I;

V_o=V_o+offset;

end

== matlab function speed_modelo_motor_frenado_con_codigoC/LIM Model/Vehicle dynamics/MATLAB Function ==
  data: vel input; f output; drag input
function f = fcn(vel,drag)

if vel > 5
    f=drag;
else
    f=0;
end

== matlab function speed_modelo_motor_frenado_con_codigoC/Calculo Maximo/MATLAB Function ==
  settings: updateMethod=DISCRETE
  data: frecuencia input; maximo output; valor input; tiempo input
function maximo = fcn(frecuencia,valor,tiempo)

   persistent antiguo_maximo
    if isempty(antiguo_maximo)
       antiguo_maximo=0;
    end
    persistent t_maximo
    if isempty(t_maximo)
       t_maximo=0;
    end

periodo=1/abs(frecuencia);


if abs(valor)>=antiguo_maximo
    maximo=abs(valor);
    antiguo_maximo=abs(valor);
    t_maximo=tiempo;
else
    maximo=antiguo_maximo;
    if tiempo>t_maximo+periodo
        maximo=abs(valor);
        antiguo_maximo=abs(valor);
        t_maximo=tiempo;
    end
end
